simulink model "RCAM_MODEL"  (R2024a)
settings: Solver=ode45  StartTime=0.0  StopTime=100  MaxStep=0.01  RelTol=1e-6
values from neighbouring files (symbols this model uses):
  u1max = 25*pi/180    (= 0.436332312999)    [initializeSimulation.m]    (also in rcam_initializaton.m)
  u1min = -25*pi/180    (= -0.436332312999)    [initializeSimulation.m]    (also in rcam_initializaton.m)
  u2max = 10*pi/180    (= 0.174532925199)    [initializeSimulation.m]    (also in rcam_initializaton.m)
  u2min = -25*pi/180    (= -0.436332312999)    [initializeSimulation.m]    (also in rcam_initializaton.m)
  u3max = 30*pi/180    (= 0.523598775598)    [initializeSimulation.m]    (also in rcam_initializaton.m)
  u3min = -30*pi/180    (= -0.523598775598)    [initializeSimulation.m]    (also in rcam_initializaton.m)
  u4max = 10*pi/180    (= 0.174532925199)    [initializeSimulation.m]    (also in rcam_initializaton.m)
  u4min = 0    [initializeSimulation.m]    (also in rcam_initializaton.m)
  u5max = 10*pi/180    (= 0.174532925199)    [initializeSimulation.m]    (also in rcam_initializaton.m)
  u5min = 0    [initializeSimulation.m]    (also in rcam_initializaton.m)
  x0 = Xstar    [initializeSimulation.m]    (also in rcam_initializaton.m = [85.0)
  Xgeodetic0 = [lat0;long0;h0]    [initializeSimulation.m]
undefined symbols (not defined in the file or in its folder): rcam_model
libraries: aerolibfltsims x2, sharedtransform x1, shared6dof x1
settings Model: Creator=ragup  LastModifiedBy=ragup

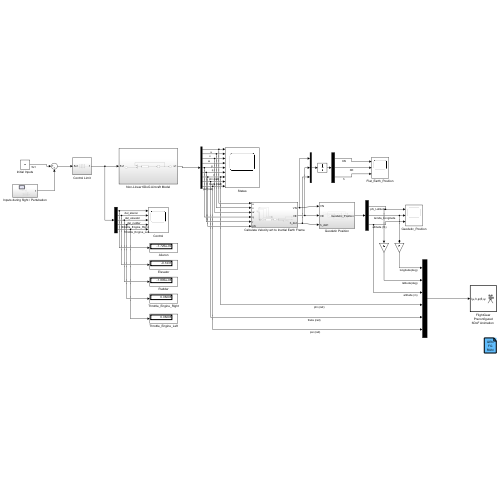
[thumbnail: Simulink's stored preview of the top-level diagram]
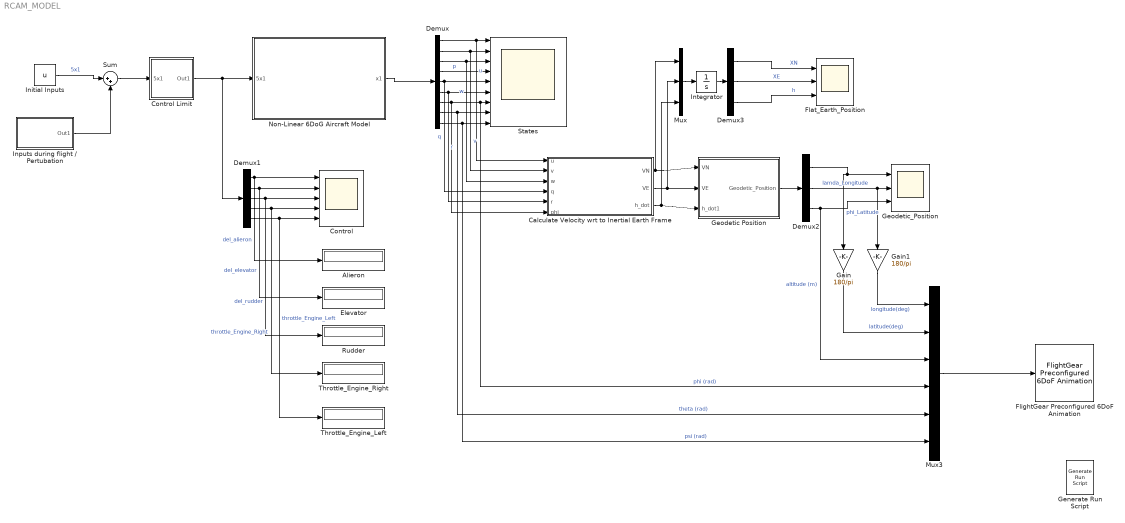
== system RCAM_MODEL ==
  Alieron : Display
  Calculate Velocity wrt to Inertial Earth Frame : Subsystem
  Control : Scope  NumInputPorts=5
  Control Limit : Subsystem
  Demux : Demux  Outputs=9
  Demux1 : Demux  Outputs=5
  Demux2 : Demux  Outputs=3
  Demux3 : Demux  Outputs=3
  Elevator : Display
  Flat_Earth_Position : Scope  NumInputPorts=3
  "FlightGear Preconfigured 6DoF Animation " : aerolibfltsims/FlightGear Preconfigured 6DoF Animation  xFlightGearVersion=v2019.1  DestinationIpAddress=127.0.0.1  DestinationPort=5502  SampleTime=1/30  packetVersion=24
  Gain : Gain  Gain=180/pi
  Gain1 : Gain  Gain=180/pi
  Generate Run Script : aerolibfltsims/Generate Run Script  Architecture=Win64  dataFlow=Send  GeometryModelName=c172p  AirportId=BIKF  RunwayId=10  InitialAltitude=7224  InitialHeading=113  OffsetDistance=4.72  OffsetAzimuth=0  InstallScenery=off  DisableShaders=on  OriginAddress=127.0.0.1  DestinationPort=5502  OriginPort=5505  LocalAddress=127.0.0.1  OutputFileName=runfg.bat  FlightGearBaseDirectory=C:\Program Files\FlightGear 2020.3
  Geodetic Position : Subsystem
  Geodetic_Position : Scope  NumInputPorts=3
  Initial Inputs : Constant  Value=u
  Inputs during flight / Pertubation : Subsystem
  Integrator : Integrator
  Mux : Mux  Inputs=3
  Mux3 : Mux  Inputs=6
  Non-Linear 6DoG Aircraft Model : Subsystem
  Rudder : Display
  States : Scope  NumInputPorts=9
  Sum : Sum  Inputs=|++
  Throttle_Engine_Left : Display
  Throttle_Engine_Right : Display
  wires:
  Demux/1 -> Calculate Velocity wrt to Inertial Earth Frame/1(u), States/1  "u"
  Demux/2 -> Calculate Velocity wrt to Inertial Earth Frame/2(v), States/2  "v"
  Demux/3 -> Calculate Velocity wrt to Inertial Earth Frame/3(w), States/3  "w"
  Demux/4 -> States/4  "p"
  Demux/5 -> Calculate Velocity wrt to Inertial Earth Frame/4(q), States/5  "q"
  Demux/6 -> Calculate Velocity wrt to Inertial Earth Frame/5(r), States/6  "r"
  Demux1/1 -> Alieron/1, Control/1  "del_alieron"
  Demux1/2 -> Elevator/1, Control/2  "del_elevator"
  Demux1/3 -> Rudder/1, Control/3  "del_rudder"
  Demux1/4 -> Throttle_Engine_Right/1, Control/4  "throttle_Engine_Right"
  Demux1/5 -> Throttle_Engine_Left/1, Control/5  "throttle_Engine_Left"
  Non-Linear 6DoG Aircraft Model/1(x1) -> Demux/1
  Control Limit/1(Out1) -> Demux1/1, Non-Linear 6DoG Aircraft Model/1(5x1)
  Sum/1 -> Control Limit/1(5x1)
  Initial Inputs/1 -> Sum/1  "5x1"
  Inputs during flight / Pertubation/1(Out1) -> Sum/2
  Calculate Velocity wrt to Inertial Earth Frame/1(VN) -> Mux/1, Geodetic Position/1(VN)
  Calculate Velocity wrt to Inertial Earth Frame/2(VE) -> Mux/2, Geodetic Position/2(VE)
  Calculate Velocity wrt to Inertial Earth Frame/3(h_dot) -> Geodetic Position/3(h_dot1), Mux/3
  Geodetic Position/1(Geodetic_Position) -> Demux2/1
  Demux2/1 -> Geodetic_Position/1, Gain/1  "phi_Latitude"
  Demux2/2 -> Gain1/1, Geodetic_Position/2  "lamda_Longitude"
  Demux3/3 -> Flat_Earth_Position/3  "h"
  Demux3/2 -> Flat_Earth_Position/2  "XE"
  Demux3/1 -> Flat_Earth_Position/1  "XN"
  Mux/1 -> Integrator/1
  Integrator/1 -> Demux3/1
  Mux3/1 -> "FlightGear Preconfigured 6DoF Animation "/1
  Gain1/1 -> Mux3/1  "longitude(deg)"
  Gain/1 -> Mux3/2  "latitude(deg)"
  Demux2/3 -> Mux3/3, Geodetic_Position/3  "altitude (m)"
  Demux/7 -> Calculate Velocity wrt to Inertial Earth Frame/6(phi), States/7, Mux3/4  "phi (rad)"
  Demux/8 -> Mux3/5, States/8  "theta (rad)"
  Demux/9 -> States/9, Mux3/6  "psi (rad)"

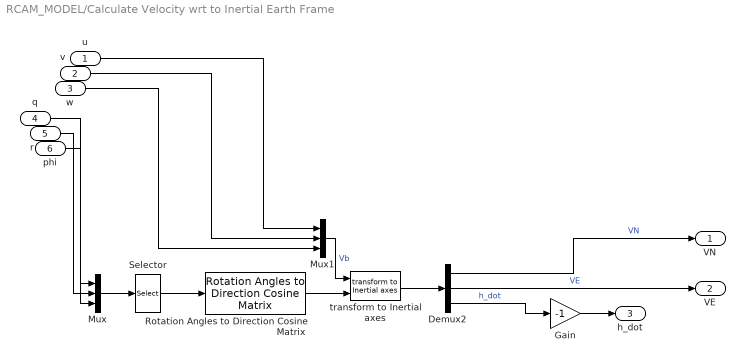
== system RCAM_MODEL/Calculate Velocity wrt to Inertial Earth Frame ==
  u : Inport
  v : Inport  Port=2
  w : Inport  Port=3
  q : Inport  Port=4
  r : Inport  Port=5
  phi : Inport  Port=6
  Demux2 : Demux  Outputs=3
  Gain : Gain  Gain=-1
  Mux : Mux  Inputs=3
  Mux1 : Mux  Inputs=3
  Rotation Angles to Direction Cosine Matrix : sharedtransform/Rotation Angles to Direction Cosine Matrix  rotationOrder=ZYX  aMode=aMode
  Selector : Selector  InputPortWidth=3  IndexOptions=Index vector (dialog)  Indices=[3 2 1]  OutputSizes=1
  "transform to Inertial axes " : shared6dof/6DOF (Euler Angles)/transform to Inertial axes   SystemSampleTime=-1  VariantActivationTime=update diagram  AllowFlexibleInterface=on  Latency=0  AutoFrameSizeCalculation=off
  VN : Outport
  VE : Outport  Port=2
  h_dot : Outport  Port=3
  wires:
  "transform to Inertial axes "/1 -> Demux2/1
  phi/1 -> Mux/3
  Mux/1 -> Selector/1
  Selector/1 -> Rotation Angles to Direction Cosine Matrix/1
  Demux2/2 -> VE/1  "VE"
  Rotation Angles to Direction Cosine Matrix/1 -> "transform to Inertial axes "/2
  Mux1/1 -> "transform to Inertial axes "/1  "Vb"
  w/1 -> Mux1/3
  r/1 -> Mux/2
  Demux2/1 -> VN/1  "VN"
  q/1 -> Mux/1
  u/1 -> Mux1/1
  v/1 -> Mux1/2
  Demux2/3 -> Gain/1  "h_dot"
  Gain/1 -> h_dot/1

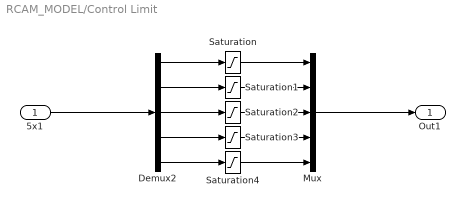
== system RCAM_MODEL/Control Limit ==
  5x1 : Inport
  Demux2 : Demux  Outputs=5
  Mux : Mux  Inputs=5
  Saturation : Saturate  UpperLimit=u1max  LowerLimit=u1min
  Saturation1 : Saturate  UpperLimit=u2max  LowerLimit=u2min
  Saturation2 : Saturate  UpperLimit=u3max  LowerLimit=u3min
  Saturation3 : Saturate  UpperLimit=u4max  LowerLimit=u4min
  Saturation4 : Saturate  UpperLimit=u5max  LowerLimit=u5min
  Out1 : Outport
  wires:
  Demux2/4 -> Saturation3/1
  Saturation2/1 -> Mux/3
  Saturation3/1 -> Mux/4
  Saturation4/1 -> Mux/5
  Demux2/1 -> Saturation/1
  Saturation/1 -> Mux/1
  Demux2/2 -> Saturation1/1
  Demux2/5 -> Saturation4/1
  Saturation1/1 -> Mux/2
  Demux2/3 -> Saturation2/1
  5x1/1 -> Demux2/1
  Mux/1 -> Out1/1

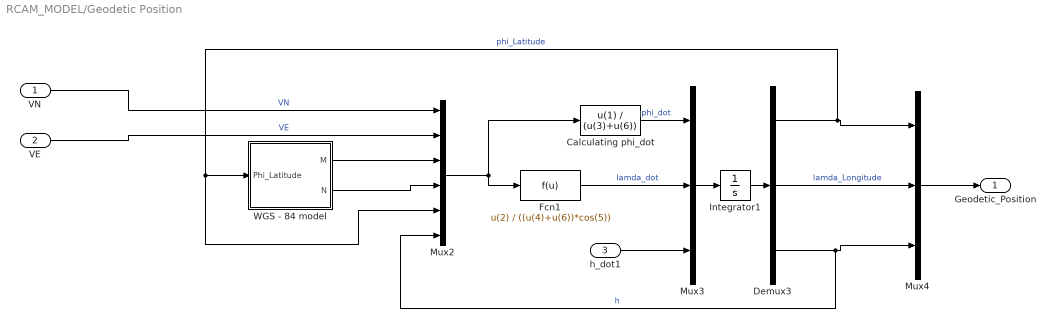
== system RCAM_MODEL/Geodetic Position ==
  VN : Inport
  VE : Inport  Port=2
  h_dot1 : Inport  Port=3
  Calculating phi_dot : Fcn  Expr=u(1) / (u(3)+u(6))
  Demux3 : Demux  Outputs=3
  Fcn1 : Fcn  Expr=u(2) / ((u(4)+u(6))*cos(5))
  Integrator1 : Integrator  InitialCondition=Xgeodetic0
  Mux2 : Mux  Inputs=6
  Mux3 : Mux  Inputs=3
  Mux4 : Mux  Inputs=3
  WGS - 84 model : Subsystem
  Geodetic_Position : Outport
  wires:
  Fcn1/1 -> Mux3/2  "lamda_dot"
  Mux3/1 -> Integrator1/1
  Integrator1/1 -> Demux3/1
  Demux3/3 -> Mux2/6, Mux4/3  "h"
  Mux2/1 -> Fcn1/1, Calculating phi_dot/1
  Demux3/1 -> WGS - 84 model/1(Phi_Latitude), Mux2/5, Mux4/1  "phi_Latitude"
  Mux4/1 -> Geodetic_Position/1
  Calculating phi_dot/1 -> Mux3/1  "phi_dot"
  Demux3/2 -> Mux4/2  "lamda_Longitude"
  VE/1 -> Mux2/2  "VE"
  VN/1 -> Mux2/1  "VN"
  h_dot1/1 -> Mux3/3
  WGS - 84 model/2(N) -> Mux2/4
  WGS - 84 model/1(M) -> Mux2/3

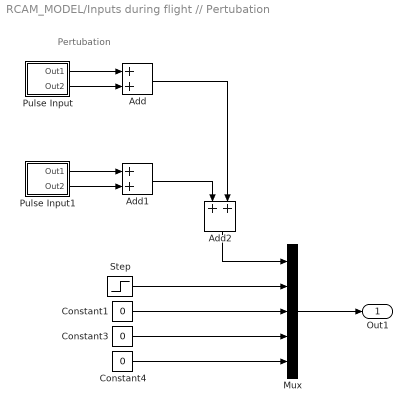
== system RCAM_MODEL/Inputs during flight // Pertubation ==
  note: Pertubation
  Add : Sum
  Add1 : Sum
  Add2 : Sum
  Constant1 : Constant  Value=0
  Constant3 : Constant  Value=0
  Constant4 : Constant  Value=0
  Mux : Mux  Inputs=5
  Pulse Input : Subsystem
  Pulse Input1 : Subsystem
  Step : Step  Time=100  After=2*pi/180  SampleTime=0
  Out1 : Outport
  wires:
  Pulse Input/1(Out1) -> Add/1
  Pulse Input/2(Out2) -> Add/2
  Constant1/1 -> Mux/3
  Mux/1 -> Out1/1
  Pulse Input1/1(Out1) -> Add1/1
  Pulse Input1/2(Out2) -> Add1/2
  Add1/1 -> Add2/1
  Add/1 -> Add2/2
  Add2/1 -> Mux/1
  Step/1 -> Mux/2
  Constant3/1 -> Mux/4
  Constant4/1 -> Mux/5

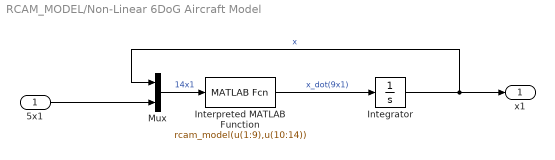
== system RCAM_MODEL/Non-Linear 6DoG Aircraft Model ==
  5x1 : Inport
  Integrator : Integrator  InitialCondition=x0
  Interpreted MATLAB Function : MATLABFcn  MATLABFcn=rcam_model(u(1:9),u(10:14))
  Mux : Mux  Inputs=2
  x1 : Outport
  wires:
  Interpreted MATLAB Function/1 -> Integrator/1  "x_dot(9x1)"
  Integrator/1 -> Mux/1, x1/1  "x"
  Mux/1 -> Interpreted MATLAB Function/1  "14x1"
  5x1/1 -> Mux/2

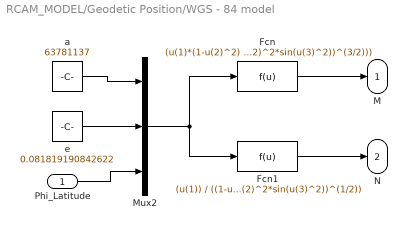
== system RCAM_MODEL/Geodetic Position/WGS - 84 model ==
  Phi_Latitude : Inport
  Fcn : Fcn  Expr=(u(1)*(1-u(2)^2) / ((1-u(2)^2*sin(u(3)^2))^(3/2)))
  Fcn1 : Fcn  Expr=(u(1)) / ((1-u(2)^2*sin(u(3)^2))^(1/2))
  Mux2 : Mux  Inputs=3
  a : Constant  Value=63781137
  e : Constant  Value=0.081819190842622
  M : Outport
  N : Outport  Port=2
  wires:
  a/1 -> Mux2/1
  e/1 -> Mux2/2
  Fcn1/1 -> N/1
  Mux2/1 -> Fcn1/1, Fcn/1
  Phi_Latitude/1 -> Mux2/3
  Fcn/1 -> M/1

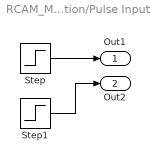
== system RCAM_MODEL/Inputs during flight // Pertubation/Pulse Input ==
  Step : Step  Time=20  After=5*pi/180  SampleTime=0
  Step1 : Step  Time=20+10  After=-5*pi/180  SampleTime=0
  Out1 : Outport
  Out2 : Outport  Port=2
  wires:
  Step/1 -> Out1/1
  Step1/1 -> Out2/1

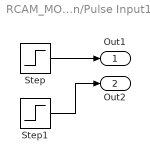
== system RCAM_MODEL/Inputs during flight // Pertubation/Pulse Input1 ==
  Step : Step  Time=50  After=-5*pi/180  SampleTime=0
  Step1 : Step  Time=50+10  After=5*pi/180  SampleTime=0
  Out1 : Outport
  Out2 : Outport  Port=2
  wires:
  Step1/1 -> Out2/1
  Step/1 -> Out1/1
